simulink model "reclaim_prototype_control"  (R2024a)
settings: Solver=FixedStepAuto  StartTime=0.0  StopTime=10.0  FixedStep=0.001  RelTol=1e-3
settings Model: Creator=shadysiam  LastModifiedBy=shadysiam

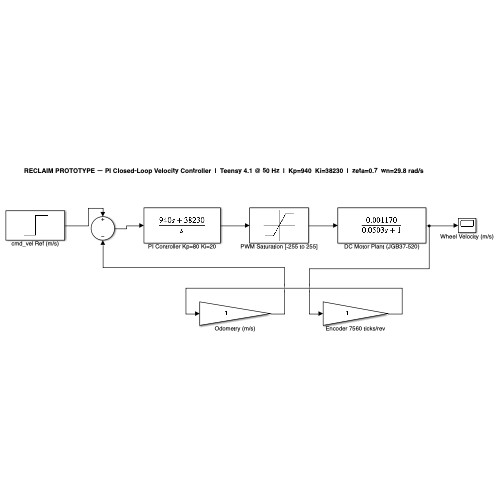
[thumbnail: Simulink's stored preview of the top-level diagram]
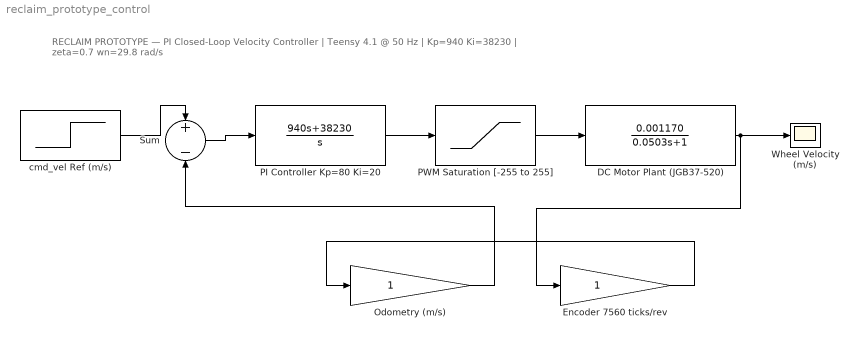
== system reclaim_prototype_control ==
  note: RECLAIM PROTOTYPE — PI Closed-Loop Velocity Controller | Teensy 4.1 @ 50 Hz | Kp=940 Ki=38230 | zeta=0.7 wn=29.8 rad/s
  DC Motor Plant (JGB37-520) : TransferFcn  Numerator=[0.001170]  Denominator=[0.0503 1]
  Encoder 7560 ticks/rev : Gain
  Odometry (m/s) : Gain
  PI Controller Kp=80 Ki=20 : TransferFcn  Numerator=[940 38230]  Denominator=[1 0]
  PWM Saturation [-255 to 255] : Saturate  UpperLimit=255  LowerLimit=-255
  Sum : Sum  Inputs=+-
  Wheel Velocity (m/s) : Scope
  cmd_vel Ref (m/s) : Step  Time=0.5  After=0.20  SampleTime=0
  wires:
  cmd_vel Ref (m/s)/1 -> Sum/1
  Sum/1 -> PI Controller Kp=80 Ki=20/1
  PI Controller Kp=80 Ki=20/1 -> PWM Saturation [-255 to 255]/1
  PWM Saturation [-255 to 255]/1 -> DC Motor Plant (JGB37-520)/1
  DC Motor Plant (JGB37-520)/1 -> Wheel Velocity (m/s)/1, Encoder 7560 ticks/rev/1
  Encoder 7560 ticks/rev/1 -> Odometry (m/s)/1
  Odometry (m/s)/1 -> Sum/2
